simulink model "TargetModel_Pascal"  (R2014a)
settings: Solver=ode3  SolverMode=SingleTasking  StartTime=0.0  StopTime=Inf  FixedStep=0.1  RelTol=1e-3
PostLoadFcn:
  | loadRobotParameters
  | 
  | allotedRunTime = 3*60; % [sec] Time allowed for run
  | 
  | % starting parameters
  | % The timer starts once the robot has moved a certain distance from the
  | % starting point
  | startPos = [50 50]; % [cm]
  | startingRadius = 10; % [cm]
  | 
  | % Target parameters
  | targetBoundaryRadius = 7; % [cm] radius considered at location
  | statTimeReq = 2.5; % [sec] minimum time robot must be at location
InitFcn:
  | close('all','force');
StartFcn:
  | %reset(SimDisplay.getInstance());
undefined symbols (not defined in the file or in its folder): AxleLength, dT, EncRes, TargetPositions, WheelRadius
libraries: arduinolib x5, simulink x1
CloseFcn:
  | close('all','force');
settings Model: SimulationMode=external  PauseTimes=14  ExtModeTrigDuration=2  Creator=gpacitti  LastModifiedBy=planger
settings DataIOCC: SignalLoggingSaveFormat=ModelDataLogs  SaveOutput=off  SignalLogging=off  DSMLogging=off  SaveTime=off
settings OptimizationCC: ExpressionDepthLimit=2147483647  OptimizeModelRefInitCode=on  LifeSpan=Inf
settings DebuggingCC: UnderspecifiedInitializationDetection=Classic  SolverPrmCheckMsg=none  MultiTaskDSMMsg=warning  MultiTaskCondExecSysMsg=none  ParameterPrecisionLossMsg=none  StateNameClashWarn=warning
settings HardwareCC: ProdLargestAtomicInteger=Long  ProdLargestAtomicFloat=Double  ProdEndianess=LittleEndian  ProdHWDeviceType=ARM Compatible->ARM Cortex
settings RTWCC: SystemTargetFile=realtime.tlc  GenerateMakefile=off  TemplateMakefile=realtime.tmf  Description=Run on Target Hardware  RTWVerbose=off  ProcessScript=realtime_make_rtw_hook  IncludeERTFirstTime=on
settings CodeAppCC: CustomSymbolStrType=$N$R$M  InternalIdentifier=Classic
settings STFCustomTargetCC: TargetLibSuffix=.a  GenerateSampleERTMain=on  ConcurrentExecutionCompliant=off  GeneratePreprocessorConditionals=Use local settings  ERTCustomFileBanners=on  SupportNonInlinedSFcns=off  SupportVariableSizeSignals=on  MATLABClassNameForMDSCustomization=Simulink.SoftwareTarget.ERTCustomization  GRTInterface=off  SystemTargetFile=realtime.tlc
settings ERTTargetCC: CombineOutputUpdateFcns=off  SupportContinuousTime=on  SupportVariableSizeSignals=on  ExtMode=on  ExtModeTransport=3  ExtModeMexFile=ext_serial_win32_comm  ExtModeMexArgs=0 17 115200 30  ERTSrcFileBannerTemplate=realtime_code_template.cgt  ERTHdrFileBannerTemplate=realtime_code_template.cgt  ERTDataSrcFileTemplate=realtime_code_template.cgt  ERTDataHdrFileTemplate=realtime_code_template.cgt  ERTCustomFileTemplate=realtime_file_process.tlc
settings ConfigComp: Description=Design Verifier Custom Configuration Component  DVMaxTestCaseSteps=500  DVTestSuiteOptimization=CombinedObjectives (Nonlinear Extended)

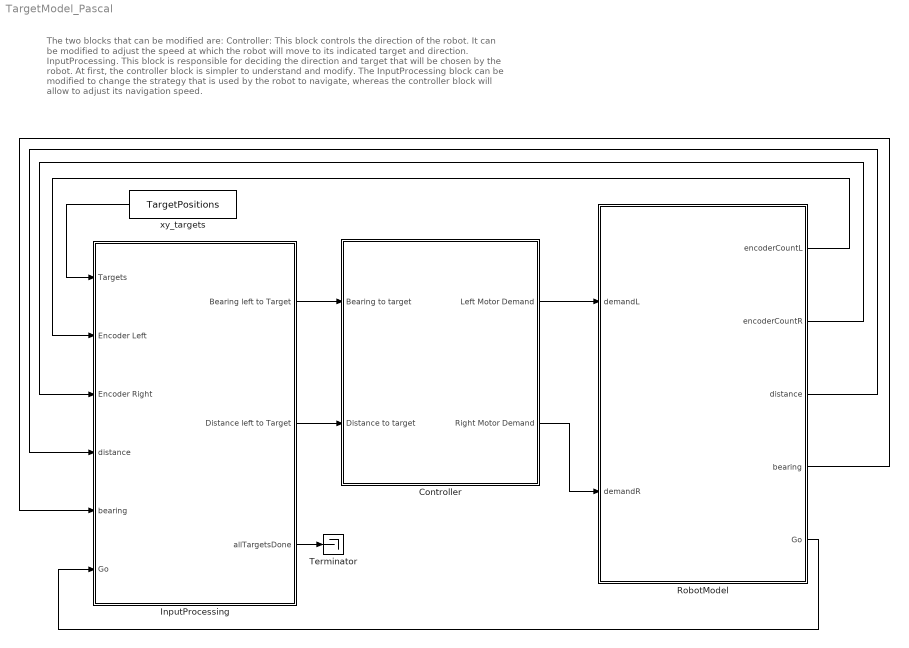
== system TargetModel_Pascal ==
  note: The two blocks that can be modified are:
      | Controller: This block controls the direction of the robot. It can be modified to adjust the speed at which the robot will move to its indicated target and direction.
      | InputProcessing. This block is responsible for deciding the direction and target that will be chosen by the robot.
      |
      | At first, the controller block is simpler to understand and modify.
      | The InputProcessing block can be modified to change the strategy that is used by the robot to navigate, whereas the controller block will allow to adjust its navigation speed.
  Controller : Subsystem  TreatAsAtomicUnit=on
      mask Display: image('Arduino_Mega_2560.jpg',[0.75/2,0.3,0.25,0.4]);
  InputProcessing : Subsystem
      mask Display: image('Arduino_Mega_2560.jpg',[0.75/2,0.3,0.25,0.3]);
  RobotModel : Subsystem
      mask Display: image('robot_3d.jpg',[0.20,0.3,0.45,0.3]);
  Terminator : Terminator
  xy_targets : Constant  Value=TargetPositions  OutDataTypeStr=single  SampleTime=1
  wires:
  RobotModel/2(encoderCountR) -> InputProcessing/3(Encoder Right)
  RobotModel/1(encoderCountL) -> InputProcessing/2(Encoder Left)
  xy_targets/1 -> InputProcessing/1(Targets)
  InputProcessing/2(Distance left to Target) -> Controller/2(Distance to target)
  InputProcessing/1(Bearing left to Target) -> Controller/1(Bearing to target)
  Controller/1(Left Motor Demand) -> RobotModel/1(demandL)
  Controller/2(Right Motor Demand) -> RobotModel/2(demandR)
  RobotModel/3(distance) -> InputProcessing/4(distance)
  RobotModel/4(bearing) -> InputProcessing/5(bearing)
  RobotModel/5(Go) -> InputProcessing/6(Go)
  InputProcessing/3(allTargetsDone) -> Terminator/1

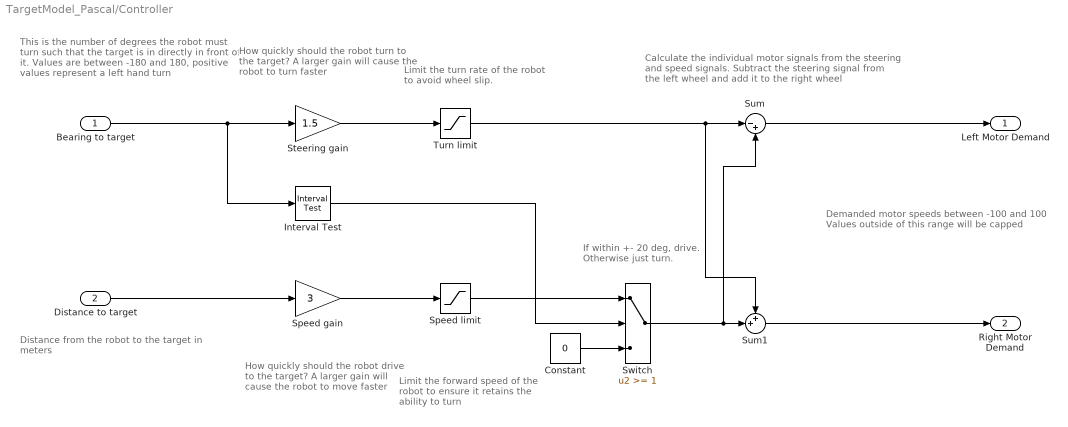
== system TargetModel_Pascal/Controller ==
  note: This is the number of degrees the robot
      | must turn such that the target is in directly
      | in front of it.
      | Values are between -180 and 180,
      | positive values represent a left hand turn
  note: Distance from the robot to the target
      | in meters
  note: Demanded motor speeds between -100 and 100
      | Values outside of this range will be capped
  note: How quickly should the robot turn
      | to the target? A larger gain will
      |  cause the robot to turn faster
  note: How quickly should the robot
      | drive to the target? A larger gain
      | will cause the robot to move
      | faster
  note: Limit the forward speed of the
      | robot to ensure it retains the
      | ability to turn
  note: Calculate the individual motor signals from the
      | steering and speed signals. Subtract the steering
      | signal from the left wheel and add it to the right
      | wheel
  note: If within +- 20 deg, drive.
      | Otherwise just turn.
  note: Limit the turn rate of the
      | robot to avoid wheel slip.
  Bearing to target : Inport  OutDataTypeStr=single
  Distance to target : Inport  Port=2  PortDimensions=1  SampleTime=dT
  Constant : Constant  Value=0  OutDataTypeStr=single
  Interval Test : simulink/Logic and Bit Operations/Interval Test  IntervalClosedRight=on  uplimit=20  IntervalClosedLeft=on  lowlimit=-20  OutDataTypeStr=boolean
      settings: AttributesFormatString=|
      | Upper = %<uplimit>
      | Lower = %<lowlimit>
  Speed gain : Gain  Gain=3
  Speed limit : Saturate  UpperLimit=50  LowerLimit=0
      settings: AttributesFormatString=|
      | Upper = %<UpperLimit>
      | Lower = %<LowerLimit>
  Steering gain : Gain  Gain=1.5
  Sum : Sum  Inputs=|-+
  Sum1 : Sum  Inputs=++|
  Switch : Switch  Threshold=1
  Turn limit : Saturate  UpperLimit=50  LowerLimit=-50
      settings: AttributesFormatString=|
      | Upper = %<UpperLimit>
      | Lower = %<LowerLimit>
  Left Motor Demand : Outport  OutDataTypeStr=single
  Right Motor Demand : Outport  Port=2  OutDataTypeStr=single
  wires:
  Speed limit/1 -> Switch/1
  Turn limit/1 -> Sum1/1, Sum/1
  Constant/1 -> Switch/3
  Interval Test/1 -> Switch/2
  Bearing to target/1 -> Steering gain/1, Interval Test/1
  Switch/1 -> Sum1/2, Sum/2
  Sum/1 -> Left Motor Demand/1
  Sum1/1 -> Right Motor Demand/1
  Speed gain/1 -> Speed limit/1
  Steering gain/1 -> Turn limit/1
  Distance to target/1 -> Speed gain/1

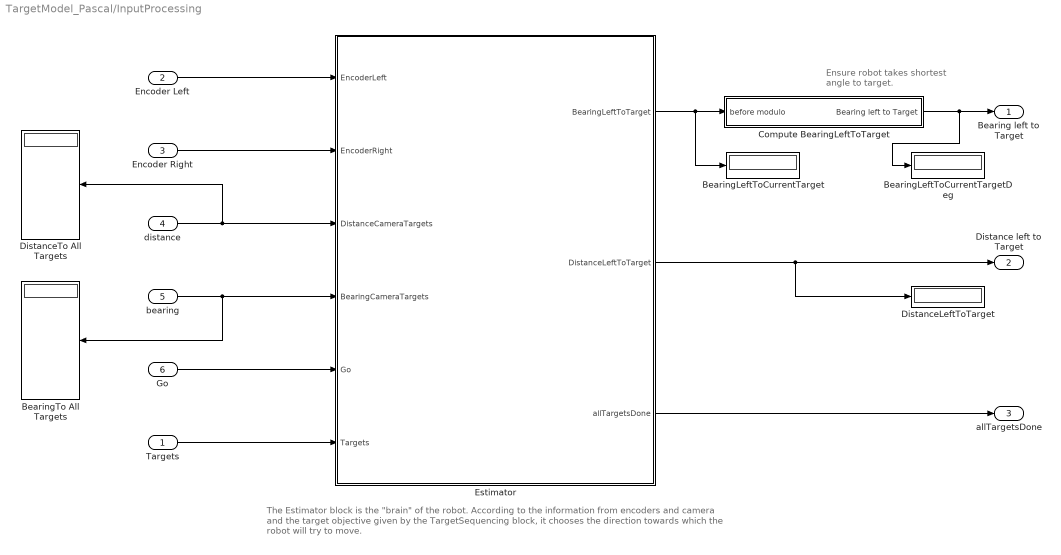
== system TargetModel_Pascal/InputProcessing ==
  note: The Estimator block is the "brain" of the robot. According to the information from encoders and camera and the
      | target objective given by the TargetSequencing block, it chooses the direction towards which the robot
      | will try to move.
  note: Ensure robot takes shortest
      | angle to target.
  Targets : Inport
  Encoder Left : Inport  Port=2  OutDataTypeStr=class(intEncoder(0))
  Encoder Right : Inport  Port=3  OutDataTypeStr=class(intEncoder(0))
  distance : Inport  Port=4
  bearing : Inport  Port=5
  Go : Inport  Port=6
  BearingLeftToCurrentTarget : Display
  BearingLeftToCurrentTargetDeg : Display
  BearingTo All Targets : Display
  Compute BearingLeftToTarget : Subsystem
  DistanceLeftToTarget : Display
  DistanceTo All Targets : Display
  Estimator : Stateflow chart  TreatAsAtomicUnit=on
  Bearing left to Target : Outport  SampleTime=dT
  Distance left to Target : Outport  Port=2
  allTargetsDone : Outport  Port=3
  wires:
  distance/1 -> DistanceTo All Targets/1, Estimator/3(DistanceCameraTargets)
  bearing/1 -> BearingTo All Targets/1, Estimator/4(BearingCameraTargets)
  Compute BearingLeftToTarget/1(Bearing left to Target) -> BearingLeftToCurrentTargetDeg/1, Bearing left to Target/1
  Estimator/2(DistanceLeftToTarget) -> DistanceLeftToTarget/1, Distance left to Target/1
  Estimator/1(BearingLeftToTarget) -> Compute BearingLeftToTarget/1(before modulo), BearingLeftToCurrentTarget/1
  Encoder Right/1 -> Estimator/2(EncoderRight)
  Encoder Left/1 -> Estimator/1(EncoderLeft)
  Targets/1 -> Estimator/6(Targets)
  Go/1 -> Estimator/5(Go)
  Estimator/3(allTargetsDone) -> allTargetsDone/1

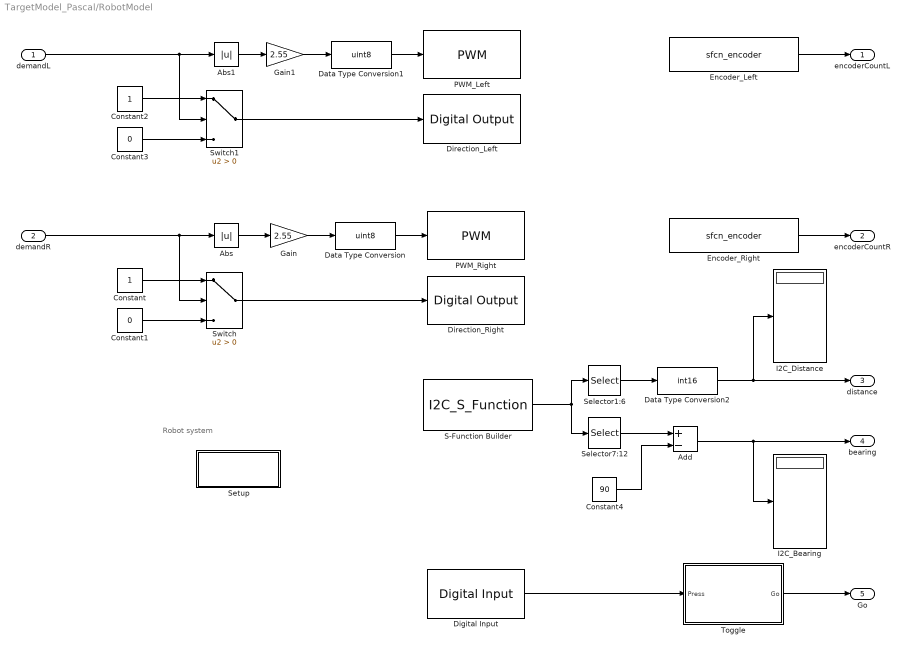
== system TargetModel_Pascal/RobotModel ==
  note: Robot system
  demandL : Inport  SampleTime=0
  demandR : Inport  Port=2  SampleTime=0
  Abs : Abs
  Abs1 : Abs
  Add : Sum  Inputs=+-  OutDataTypeStr=int8
  Constant : Constant  OutDataTypeStr=uint8
  Constant1 : Constant  Value=0  OutDataTypeStr=uint8
  Constant2 : Constant  OutDataTypeStr=uint8
  Constant3 : Constant  Value=0  OutDataTypeStr=uint8
  Constant4 : Constant  Value=90  OutDataTypeStr=uint8
  Data Type Conversion : DataTypeConversion  OutDataTypeStr=uint8  SaturateOnIntegerOverflow=on
  Data Type Conversion1 : DataTypeConversion  OutDataTypeStr=uint8  SaturateOnIntegerOverflow=on
  Data Type Conversion2 : DataTypeConversion  OutDataTypeStr=int16  SaturateOnIntegerOverflow=on
  Digital Input : arduinolib/Digital Input  pinNumber=17  sampleTime=0.1
  Direction_Left : arduinolib/Digital Output  pinNumber=7
  Direction_Right : arduinolib/Digital Output  pinNumber=4
  Encoder_Left : S-Function  InitFcn=try, set_param(gcb,'FunctionName','sfcn_encoder'), end  FunctionName=sfcn_encoder  Parameters=uint8(1),uint8(18),uint8(19)  SFunctionModules=sfcn_encoder_wrapper  EnableBusSupport=off  mask(S-Function Builder){}
      mask init:
      | val = [[.9  0.75 0.75 1 1 .9 .9 1]',[1 1 0.75 0.75 .9 .9 1 .9]'];try , sys = get_param(gcb,'SfunBuilderFcnName');if isempty(sys), sys = get_param(gcb,'FunctionName'); end,catch, sys = get_param(gcb,'FunctionName'); end
      settings: CopyFcn=set_param(gcbh,'LinkStatus','none')  PreSaveFcn=try, set_param(gcb,'FunctionName','sfcn_encoder'), end  OpenFcn=sfunctionwizard(gcbh)
      mask Display: plot(val(:,1),val(:,2)),disp(sys), port_label('output',1,'pos')
  Encoder_Right : S-Function  InitFcn=try, set_param(gcb,'FunctionName','sfcn_encoder'), end  FunctionName=sfcn_encoder  Parameters=uint8(2),uint8(2),uint8(3)  SFunctionModules=sfcn_encoder_wrapper  EnableBusSupport=off  mask(S-Function Builder){}
      mask init: same as TargetModel_Pascal/RobotModel/Encoder_Left
      settings: CopyFcn=set_param(gcbh,'LinkStatus','none')  PreSaveFcn=try, set_param(gcb,'FunctionName','sfcn_encoder'), end  OpenFcn=sfunctionwizard(gcbh)
      mask Display: plot(val(:,1),val(:,2)),disp(sys), port_label('output',1,'pos')
  Gain : Gain  Gain=2.55
  Gain1 : Gain  Gain=2.55
  I2C_Bearing : Display
  I2C_Distance : Display
  PWM_Left : arduinolib/PWM  pinNumber=6
  PWM_Right : arduinolib/PWM  pinNumber=5
  S-Function Builder : S-Function  InitFcn=try, set_param(gcb,'FunctionName','I2C_S_Function'), end  FunctionName=I2C_S_Function  Parameters=uint8(1)  SFunctionModules=I2C_S_Function_wrapper  EnableBusSupport=off  mask(S-Function Builder){}
      mask help: Simulink:masks:SFunctionBuilder_MD
      mask init: same as TargetModel_Pascal/RobotModel/Encoder_Left
      settings: CopyFcn=set_param(gcbh,'LinkStatus','none')  PreSaveFcn=try, set_param(gcb,'FunctionName','I2C_S_Function'), end  OpenFcn=sfunctionwizard(gcbh)
      mask Display: plot(val(:,1),val(:,2)),disp(sys), port_label('input',1,'Send'), port_label('output',1,'Receive')
  Selector1:6 : Selector  InputPortWidth=12  Indices=[1:6]
  Selector7:12 : Selector  InputPortWidth=12  Indices=[7:12]
  Setup : Subsystem
  Switch : Switch  Criteria=u2 > Threshold
  Switch1 : Switch  Criteria=u2 > Threshold
  Toggle : Stateflow chart  TreatAsAtomicUnit=on
  encoderCountL : Outport  OutDataTypeStr=class(intEncoder(0))
  encoderCountR : Outport  Port=2  OutDataTypeStr=class(intEncoder(0))
  distance : Outport  Port=3
  bearing : Outport  Port=4
  Go : Outport  Port=5
  wires:
  Encoder_Right/1 -> encoderCountR/1
  Encoder_Left/1 -> encoderCountL/1
  Abs/1 -> Gain/1
  Gain/1 -> Data Type Conversion/1
  Data Type Conversion/1 -> PWM_Right/1
  Constant/1 -> Switch/1
  Constant1/1 -> Switch/3
  Switch/1 -> Direction_Right/1
  Abs1/1 -> Gain1/1
  Gain1/1 -> Data Type Conversion1/1
  Data Type Conversion1/1 -> PWM_Left/1
  Constant2/1 -> Switch1/1
  Constant3/1 -> Switch1/3
  Switch1/1 -> Direction_Left/1
  Data Type Conversion2/1 -> distance/1, I2C_Distance/1
  Add/1 -> I2C_Bearing/1, bearing/1
  demandR/1 -> Switch/2, Abs/1
  demandL/1 -> Switch1/2, Abs1/1
  Digital Input/1 -> Toggle/1(Press)
  Toggle/1(Go) -> Go/1
  S-Function Builder/1 -> Selector1:6/1, Selector7:12/1
  Selector7:12/1 -> Add/1
  Constant4/1 -> Add/2
  Selector1:6/1 -> Data Type Conversion2/1

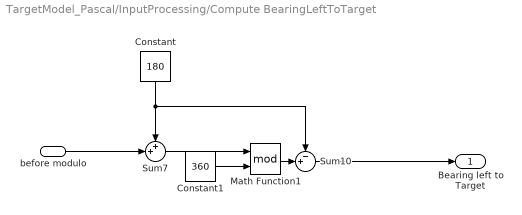
== system TargetModel_Pascal/InputProcessing/Compute BearingLeftToTarget ==
  before modulo : Inport
  Constant : Constant  Value=180  OutDataTypeStr=Inherit: Inherit via back propagation
  Constant1 : Constant  Value=360  OutDataTypeStr=Inherit: Inherit via back propagation
  Math Function1 : Math  Operator=mod  SaturateOnIntegerOverflow=on
  Sum10 : Sum  Inputs=-+|
  Sum7 : Sum  Inputs=++|
  Bearing left to Target : Outport  SampleTime=dT
  wires:
  before modulo/1 -> Sum7/2
  Sum10/1 -> Bearing left to Target/1
  Math Function1/1 -> Sum10/2
  Constant1/1 -> Math Function1/2
  Sum7/1 -> Math Function1/1
  Constant/1 -> Sum10/1, Sum7/1

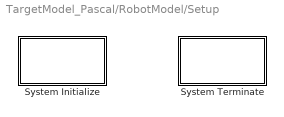
== system TargetModel_Pascal/RobotModel/Setup ==
  System Initialize : Subsystem  mask(System Initialize){ShowInLibBrowser=0}
      mask prompts: ShowInLibBrowser "Simulink:masks:CustCodeMaskParam1_MP"
      settings: CopyFcn=cccopyfcn(gcb)  OpenFcn=ccopenfcn('System Initialize Function')
      mask Help: eval('feval(''rtwprivate'',''rtwhelpview'',''rtw_sys_initialize_block'')');
      mask Display: disp('System\nInitialize');
  System Terminate : Subsystem  mask(System Terminate){ShowInLibBrowser=0}
      mask prompts: ShowInLibBrowser "Simulink:masks:CustCodeMaskParam1_MP"
      settings: CopyFcn=cccopyfcn(gcb)  OpenFcn=ccopenfcn('System Terminate Function')
      mask Help: eval('feval(''rtwprivate'',''rtwhelpview'',''rtw_sys_terminate_block'')');
      mask Display: disp('System\nTerminate');

== system TargetModel_Pascal/RobotModel/Setup/System Initialize ==

== system TargetModel_Pascal/RobotModel/Setup/System Terminate ==

== stateflow chart TargetModel_Pascal/InputProcessing/Estimator ==
  state Standby
    entry:
    %Init
    encoder_left_prev_target = int32(0);
    encoder_right_prev_target = int32(0);
    ind=uint8(0);
    CurrentDistance=single(0);
    prev_target = single(startPos);
    prev_bearing = single(0);
    TargetIndex = uint8(0);
    allTargetsDone=false;
  state Running
    state Next_Target
      entry:
      TargetIndex = TargetIndex + 1;
      %Calc relative distance to next target
      DistanceToTarget = norm(Targets(TargetIndex,1:2)-prev_target);
      %Calc relative bearing to next target
      BearingToTarget = atan2d(Targets(TargetIndex,2)-prev_target(2),...
      Targets(TargetIndex,1)-prev_target(1)) - prev_bearing;
      %Save values for relative moves
      prev_target = Targets(TargetIndex,1:2);
      prev_bearing=prev_bearing+BearingToTarget;
      encoder_left_prev_target = EncoderLeft;
      encoder_right_prev_target = EncoderRight;
      DistanceLeftToTarget = DistanceToTarget;
      BearingLeftToTarget = BearingToTarget;
    state Apply_camera_correction
      entry:
      %Find the closest match between seen targets and current destination
      TargetFound=uint8(0);
      dist_left = int16(DistanceLeftToTarget);
      for ind=1:uint8(length(DistanceCameraTargets))
      if(DistanceCameraTargets(ind) ~= 0 )
      if(abs(DistanceCameraTargets(ind) - dist_left)<10)
      if (TargetFound==0 || abs(DistanceCameraTargets(TargetFound) - ...
      dist_left)>abs(DistanceCameraTargets(ind) - dist_left))
      TargetFound=uint8(ind);
      end
      end
      end
      end
      %If a target is found update the distance and bearing from the camera
      if ( TargetFound ~= 0 )
      DistanceToTarget = single(DistanceCameraTargets(TargetFound));
      BearingToTarget = single(BearingCameraTargets(TargetFound))/2;
      encoder_left_prev_target = EncoderLeft;
      encoder_right_prev_target = EncoderRight;
      end
    state Wait_for_scoring
      entry:
      DistanceLeftToTarget = single(0);
    state Calc_next_robot_move
      entry,during:
      %Calc the new trajectory based on what has already been done
      dL = single(EncoderLeft - encoder_left_prev_target) * 2 * WheelRadius * pi / EncRes;
      dR = single(EncoderRight - encoder_right_prev_target) * 2 * WheelRadius * pi / EncRes;
      CurrentDistance = ((dL + dR)/2);
      CurrentBearing = single(((dR - dL)*180) / (AxleLength*pi));
      DistanceLeftToTarget = DistanceToTarget - CurrentDistance;
      BearingLeftToTarget = BearingToTarget - CurrentBearing;
    (default) -> Next_Target
    Next_Target -> Calc_next_robot_move
    Wait_for_scoring -> Next_Target : after(3,sec)
    Calc_next_robot_move -> Wait_for_scoring [order 1] : [DistanceLeftToTarget < 7]
    Apply_camera_correction -> Calc_next_robot_move
    Calc_next_robot_move -> Apply_camera_correction [order 2] : [CurrentDistance>5 && DistanceLeftToTarget > 20]
  state All_targets_done
    entry:
    DistanceLeftToTarget = single(0);
  state Finished
    entry:
    allTargetsDone=true;
  (default) -> Standby
  Standby -> Running : [Go == true]
  Running -> All_targets_done : [DistanceLeftToTarget < 7 && TargetIndex >= length(Targets) ]
  All_targets_done -> Finished : after(3,sec)
  data: BearingLeftToTarget output single size=1; TargetIndex local uint8 size=1 =0; EncoderLeft input int32 size=1; EncoderRight input int32 size=1; DistanceLeftToTarget output single size=1; DistanceCameraTargets input int16; TargetFound local uint8 size=1; BearingCameraTargets input int8; AxleLength parameter single size=1; WheelRadius parameter single size=1; EncRes parameter single size=1; encoder_right_prev_target local int32; ind local uint8; dR local single; dL local single; CurrentDistance local single; CurrentBearing local single; dist_left local int16; encoder_left_prev_target local int32; Go input boolean; startPos parameter; Targets input single; prev_target local single; prev_bearing local single; BearingToTarget local single; DistanceToTarget local single; allTargetsDone output boolean

== stateflow chart TargetModel_Pascal/RobotModel/Toggle ==
  state OFF
    entry: Go = false;
  state ON
    entry: Go = true;
  state Wait
  (default) -> OFF
  OFF -> Wait : [Press == 0]
  Wait -> ON : after(3,sec)
  data: Press input; Go output
